simulink model "CDCJournalModel"  (R2018b)
settings: Solver=FixedStepAuto  StartTime=0.0  StopTime=p.T  FixedStep=p.Ts  RelTol=1e-3
PreLoadFcn:
  | preLoadCallback
StartFcn:
  | startCallback
StopFcn:
  | stopCallback
values from neighbouring files (symbols this model uses):
  p = simulationParametersClass    [preLoadCallback.m]
  turbineCp = 0.5    [ARPAE30kW_ts.m]
libraries: myLibrary x17, simulink x13, lowLevel x6, controllerComponents x4, performanceIndexComponents x3, headingSetpointCaclulation x1, RLSUpdate_ul x1, dspstat3 x1
(part 2 of 2)

== system CDCJournalModel/Controller/Optimization Controller/Heading Setpoint Calculation/Detect Iteration Change ==
  In1 : Inport
  Detect Decrease : simulink/Logic and Bit Operations/Detect Decrease  vinit=0.0  OutDataTypeStr=boolean
  Out1 : Outport
  wires:
  In1/1 -> Detect Decrease/1
  Detect Decrease/1 -> Out1/1

== system CDCJournalModel/Controller/Optimization Controller/Performance Calculation/EnergyTerm ==
  vApp : Inport
  reset : Inport  Port=2
  time : Inport  Port=3
  vWind : Inport  Port=4
  Mean Energy : Subsystem  VariantControl=variantMeanEnergy
  Power Augmentation Ratio : Subsystem  VariantControl=variantPowerAugmentationRatio
  value : Outport

== system CDCJournalModel/Controller/Optimization Controller/Performance Calculation/Iteration Time Clock ==
  reset : Inport
  Clock : Clock
  Constant1 : Constant  Value=p.Ts
  If Action Subsystem : Subsystem  TreatAsAtomicUnit=on
  MinMax : MinMax  Function=max  Inputs=2
  Subtract : Sum  Inputs=-+
  timeSinceIterationStart : Outport
  wires:
  If Action Subsystem/1(Out1) -> Subtract/1
  MinMax/1 -> timeSinceIterationStart/1
  Clock/1 -> Subtract/2, If Action Subsystem/1(In1)
  reset/1 -> If Action Subsystem/Trigger
  Constant1/1 -> MinMax/1
  Subtract/1 -> MinMax/2

== system CDCJournalModel/Controller/Optimization Controller/Performance Calculation/Spatial Error Term ==
  minDistanceToPath : Inport
  iterationReset : Inport  Port=2
  time : Inport  Port=3
  Subsystem : Subsystem  VariantControl=variantSpatialError
  value : Outport

== system CDCJournalModel/Controller/Spatial ILC Controller/Find Closest Point On Path/Add And Wrap ==
  offset : Inport
  startIndex : Inport  Port=2
  Add1 : Sum
  Constant2 : Constant  Value=length(p.waypointAngles)+0.5  SampleTime=-1
  Math Function : Math  Operator=mod  SaturateOnIntegerOverflow=on
  Round : Rounding  Operator=round
  Out1 : Outport
  wires:
  offset/1 -> Add1/1
  startIndex/1 -> Add1/2
  Add1/1 -> Math Function/1
  Constant2/1 -> Math Function/2
  Math Function/1 -> Round/1
  Round/1 -> Out1/1

== system CDCJournalModel/Controller/Spatial ILC Controller/Find Closest Point On Path/Extract Waypoint Angles ==
  closestIndex : Inport
  Add4 : Sum
  Constant1 : Constant  Value=p.waypointAngles  SampleTime=-1
  Constant2 : Constant  Value=p.localSearchIndexOffsetVector  SampleTime=-1
  Selector : Selector  InputPortWidth=length(p.waypointAngles)  IndexOptions=Index vector (port)  Indices=[1 3]  OutputSizes=1
  Wrap Index : myLibrary/Wrap Index  SystemSampleTime=-1
  anglesSubset : Outport
  wires:
  Selector/1 -> anglesSubset/1
  Wrap Index/1 -> Selector/2  "waypointIndicesWraped"
  Add4/1 -> Wrap Index/1  "waypointIndicesUnwrapped"
  Constant2/1 -> Add4/2
  Constant1/1 -> Selector/1
  closestIndex/1 -> Add4/1  "indexOfClosestPoint"

== system CDCJournalModel/Controller/Spatial ILC Controller/Find Closest Point On Path/Find Minimum Distance ==
  fdbk : Inport
  wayptAzimuth : Inport  Port=2
  wayptZenith : Inport  Port=3
  Distance To Waypt : myLibrary/Distance To Waypt  SystemSampleTime=-1
  Minimum : dspstat3/Minimum  operation=minimum  fcn=Value and Index  indexBase=Zero  operateOver=Entire input  Dimension=1  InputProcessing=Columns as channels (frame based)  reset=None  roiEnable=off  roiType=Rectangles  roiPortion=Entire ROI  roiOutput=Individual statistics for each ROI  roiFlag=off  roundingMode=Floor  overflowMode=off
      settings: SourceProductName=DSP System Toolbox  SourceProductBaseCode=DS
  minDistanceToPath : Outport
  offsetFromStart : Outport  Port=2
  wires:
  Distance To Waypt/1 -> Minimum/1  "distances"
  wayptAzimuth/1 -> Distance To Waypt/2
  wayptZenith/1 -> Distance To Waypt/3
  fdbk/1 -> Distance To Waypt/1
  Minimum/2 -> offsetFromStart/1  "offsetFromStart"
  Minimum/1 -> minDistanceToPath/1  "minimumDistanceToPath"

== system CDCJournalModel/Controller/Spatial ILC Controller/Get Target Point/Select Target Point ==
  closestPointIndex : Inport
  Add : Sum
  Constant : Constant  Value=p.waypointAngles
  Constant1 : Constant  Value=p.lookAheadIndexOffset
  Constant2 : Constant  Value=p.waypointAngles
  Selector1 : Selector  InputPortWidth=p.num  IndexOptions=Index vector (port)  Indices=3  OutputSizes=1
  Selector2 : Selector  InputPortWidth=p.num  IndexOptions=Index vector (port)  Indices=3  OutputSizes=1
  Wrap Index1 : myLibrary/Wrap Index  SystemSampleTime=-1
  targetWaypointAngle : Outport
  targetWaypointIndex : Outport  Port=2
  closestWaypointAngle : Outport  Port=3
  wires:
  Constant/1 -> Selector1/1
  Constant1/1 -> Add/2
  Selector1/1 -> targetWaypointAngle/1
  Add/1 -> Wrap Index1/1
  Wrap Index1/1 -> targetWaypointIndex/1, Selector1/2  "targetedWaypointIndex"
  closestPointIndex/1 -> [closestPointIndex]
  [closestPointIndex] -> Add/1
  Constant2/1 -> Selector2/1
  [closestPointIndex] -> Selector2/2
  Selector2/1 -> closestWaypointAngle/1

== system CDCJournalModel/Controller/Spatial ILC Controller/Parse Simulation Stage/Counter ==
  In1 : Inport
  Add : Sum
  Data Type Conversion : DataTypeConversion  OutDataTypeStr=uint8
  Memory : Memory  InitialCondition=1
  Out1 : Outport  OutDataTypeStr=double
  wires:
  Add/1 -> Out1/1, Memory/1
  Memory/1 -> Add/2
  In1/1 -> Data Type Conversion/1
  Data Type Conversion/1 -> Add/1

== system CDCJournalModel/Controller/Spatial ILC Controller/Parse Simulation Stage/Detect Iteration Change ==
  In1 : Inport
  Detect Decrease : simulink/Logic and Bit Operations/Detect Decrease  vinit=0.0  OutDataTypeStr=boolean
  Out1 : Outport
  wires:
  In1/1 -> Detect Decrease/1
  Detect Decrease/1 -> Out1/1

== system CDCJournalModel/Controller/Spatial ILC Controller/Settling Phase Heading Calculation/Enabled Subsystem1 ==
  plantFeedback : Inport  OutDataTypeStr=Bus: busPlantFeedback
  targetWaypoint : Inport  Port=2  Unit=rad
  Enable : EnablePort
  Calculate Heading To Waypt : myLibrary/Heading To Waypt
  Demux : Demux  Outputs=2
  headingSetpoint : Outport  Unit=rad
  wires:
  Calculate Heading To Waypt/1 -> headingSetpoint/1
  Demux/1 -> Calculate Heading To Waypt/2
  Demux/2 -> Calculate Heading To Waypt/3
  targetWaypoint/1 -> Demux/1
  plantFeedback/1 -> Calculate Heading To Waypt/1

== system CDCJournalModel/Controller/Spatial ILC Controller/Settling Phase Heading Calculation/Log Into Vector ==
  Element : Inport
  Index : Inport  Port=2
  Assignment : Assignment  DiagnosticForDimensions=Warning  IndexOptions=Index vector (port)  Indices=1  OutputSizes=1
  Constant1 : Constant  Value=zeros(p.num,1)
  Delay : Delay  DelayLength=1  InitialConditionSource=Input port  InitialCondition=0
      settings: InputPortMap=u0,p4
  headingSetpointVec : Outport
  wires:
  Assignment/1 -> headingSetpointVec/1, Delay/1
  Element/1 -> Assignment/2
  Index/1 -> Assignment/3
  Delay/1 -> Assignment/1
  Constant1/1 -> Delay/2

== system CDCJournalModel/Plant/Fault Detection/Position Fault/Azimuth Fault ==
  note: If azimuth exceeds +/- ? deg
  theta : Inport
  Abs : Abs
  Compare To Constant : simulink/Logic and Bit Operations/Compare To Constant  relop=>=  const=(180*pi/180)  OutDataTypeStr=boolean
  fault : Outport
  wires:
  Compare To Constant/1 -> fault/1
  Abs/1 -> Compare To Constant/1
  theta/1 -> Abs/1

== system CDCJournalModel/Plant/Fault Detection/Position Fault/Radius Fault ==
  r : Inport
  Abs : Abs
  Add : Sum  Inputs=+-
  Compare To Constant : simulink/Logic and Bit Operations/Compare To Constant  relop=>=  const=0.01  OutDataTypeStr=boolean
  Divide : Product  Inputs=*/
  r Target : Constant  Value=p.initPositionGFS(1)
  fault : Outport
  wires:
  r Target/1 -> Divide/2, Add/2
  Add/1 -> Abs/1
  Compare To Constant/1 -> fault/1
  r/1 -> Add/1
  Abs/1 -> Divide/1
  Divide/1 -> Compare To Constant/1

== system CDCJournalModel/Plant/Fault Detection/Position Fault/Zenith Fault ==
  note: If zenith drops below 10 deg or goes above 80 deg.
  phi : Inport
  Abs : Abs
  Compare To Constant : simulink/Logic and Bit Operations/Compare To Constant  relop=<=  const=(10*pi/180)  OutDataTypeStr=boolean
  Compare To Constant1 : simulink/Logic and Bit Operations/Compare To Constant  relop=>=  const=(80*pi/180)  OutDataTypeStr=boolean
  Logical Operator : Logic  Operator=OR  AllPortsSameDT=off  OutDataTypeStr=boolean
  fault : Outport
  wires:
  Logical Operator/1 -> fault/1
  Abs/1 -> Compare To Constant1/1, Compare To Constant/1
  phi/1 -> Abs/1
  Compare To Constant/1 -> Logical Operator/1
  Compare To Constant1/1 -> Logical Operator/2

== system CDCJournalModel/Controller/Optimization Controller/Performance Calculation/EnergyTerm/Mean Energy ==
  vApp : Inport
  reset : Inport  Port=2
  time : Inport  Port=3
  vWind : Inport  Port=4
  Mean Energy Generation : performanceIndexComponents/Mean Energy Generation  SystemSampleTime=-1
  value : Outport
  wires:
  vApp/1 -> Mean Energy Generation/1
  reset/1 -> Mean Energy Generation/2
  time/1 -> Mean Energy Generation/3
  vWind/1 -> Mean Energy Generation/4
  Mean Energy Generation/1 -> value/1

== system CDCJournalModel/Controller/Optimization Controller/Performance Calculation/EnergyTerm/Power Augmentation Ratio ==
  vApp : Inport
  reset : Inport  Port=2
  time : Inport  Port=3
  vWind : Inport  Port=4
  PAR : performanceIndexComponents/PAR  SystemSampleTime=-1
  value : Outport
  wires:
  vApp/1 -> PAR/1
  reset/1 -> PAR/2
  time/1 -> PAR/3
  vWind/1 -> PAR/4
  PAR/1 -> value/1

== system CDCJournalModel/Controller/Optimization Controller/Performance Calculation/Iteration Time Clock/If Action Subsystem ==
  In1 : Inport
  Trigger : TriggerPort  VariantControl=Variant  PortDimensions=1
  Out1 : Outport
  wires:
  In1/1 -> Out1/1

== system CDCJournalModel/Controller/Optimization Controller/Performance Calculation/Spatial Error Term/Subsystem ==
  minDistanceToPath : Inport
  iterationReset : Inport  Port=2
  time : Inport  Port=3
  Spatial Error : performanceIndexComponents/Spatial Error  SystemSampleTime=-1
  value : Outport
  wires:
  minDistanceToPath/1 -> Spatial Error/1
  iterationReset/1 -> Spatial Error/2
  time/1 -> Spatial Error/3
  Spatial Error/1 -> value/1
